simulink library "lib_GenTools_SubMatrix"  (R2015a)
settings: Solver=ode45  StartTime=0.0  StopTime=10.0  RelTol=1e-3
settings Model: Creator=jlkratz  LastModifiedBy=jlkratz

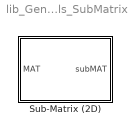
== system lib_GenTools_SubMatrix ==
  Sub-Matrix (2D) : Subsystem  mask(TSAT: Sub-Matrix (2D)){R1_M=1, R2_M=1, C1_M=1, C2_M=1, BN_M=double(gcb)}
      mask prompts: R1_M "R1_M - Starting Row Index"; R2_M "R2_M - Ending Row Index"; C1_M "C1_M - Starting Column Index"; C2_M "C2_M - Ending Column Index"; BN_M "BN_M - Block Name"
      mask help:
      | This block returns a sub-matrix within the input matrix given the row and column indices the define the sub-matrix. This block is meant for 2D matrices and will work for 1D arrays as well.
      |
      | The following restrictions apply:
      | -- MAT must be a 1-D or 2-D array
      | -- R1_M and R2_M must be real, finite, positive integers that are less than or equal to the number of rows.
      | -- C1_M and C2_M must be real, finite, positive integers that are less than or equal to the number of columns.
      | -- R2_M >= R1_M
      | -- C2_M >= C1_M
      |
      | For more information see the block help menu.
      mask Help: web(which('GenTools_TSAT_SubMatrix.html'),'-helpbrowser')

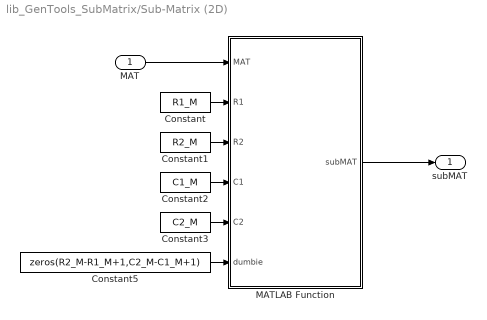
== system lib_GenTools_SubMatrix/Sub-Matrix (2D) ==
  MAT : Inport
  Constant : Constant  Value=R1_M
  Constant1 : Constant  Value=R2_M
  Constant2 : Constant  Value=C1_M
  Constant3 : Constant  Value=C2_M
  Constant5 : Constant  Value=zeros(R2_M-R1_M+1,C2_M-C1_M+1)
  MATLAB Function : MATLAB Function  TreatAsAtomicUnit=on
  subMAT : Outport
  wires:
  Constant5/1 -> MATLAB Function/6(dumbie)
  MAT/1 -> MATLAB Function/1(MAT)
  MATLAB Function/1(subMAT) -> subMAT/1
  Constant/1 -> MATLAB Function/2(R1)
  Constant1/1 -> MATLAB Function/3(R2)
  Constant2/1 -> MATLAB Function/4(C1)
  Constant3/1 -> MATLAB Function/5(C2)

== matlab function lib_GenTools_SubMatrix/Sub-Matrix (2D)/MATLAB Function ==
  data: MAT input; subMAT output; R1 input; R2 input; C1 input; C2 input; dumbie input
function subMAT  = SubMatrix2D(MAT,R1,R2,C1,C2,dumbie)
%#codegen

%Description:
%   This block returns a sub-matrix from a given matrix

%Inputs:
%   MAT - The matrix
%   R1 - Starting Row Index
%   R2 - Ending Row Index
%   C1 - Starting Column Index
%   C2 - Ending Column Index

%Outputs:
%   subMAT - The submatrix

%Calculations ------------------------------------------------------------%

subMAT = zeros(size(dumbie));
k = 1;
for i = R1:R2
    m = 1;
    for j = C1:C2
        subMAT(k,m) = MAT(i,j);
        m = m + 1;
    end
    k = k + 1;
end
